simulink model "multi_module_phase_shift_generator_base"  (R2025b)
settings: Solver=FixedStepDiscrete  StartTime=0.0  StopTime=10e3  RelTol=1e-3
settings Model: DataTypeOverride=Off  FPTShortcutValueString='{{},{''BaselineRun_2'',1,1,1,''BaselineRun_2'','''',{},''M'',''F'',''''}}'  Creator=KoayXianCong  LastModifiedBy=KoayXianCong
settings OptimizationCC: BlockReduction=off  ConditionallyExecuteInputs=off  DefaultParameterBehavior=Inlined  InheritOutputTypeSmallerThanSingle=on
settings DebuggingCC: SignalRangeChecking=warning  ArtificialAlgebraicLoopMsg=error  SingleTaskRateTransMsg=error
settings HardwareCC: ProdBitPerPointer=32.0  ProdBitPerSizeT=32.0  ProdBitPerPtrDiffT=32.0  ProdLargestAtomicFloat=None  ProdIntDivRoundTo=Undefined  ProdEndianess=Unspecified  ProdWordSize=32.0  ProdHWDeviceType=ASIC/FPGA->ASIC/FPGA  TargetBitPerPointer=64.0  TargetBitPerSizeT=64.0  TargetBitPerPtrDiffT=64.0  TargetLongLongMode=on  TargetIntDivRoundTo=Zero  TargetEndianess=LittleEndian  TargetWordSize=64.0  TargetHWDeviceType=Custom Processor->MATLAB Host Computer  ProdEqTarget=off

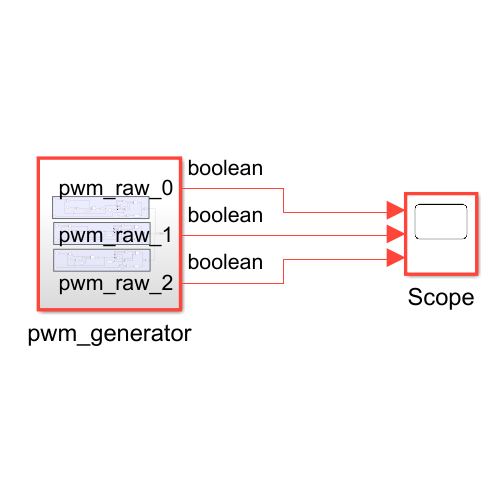
[thumbnail: Simulink's stored preview of the top-level diagram]
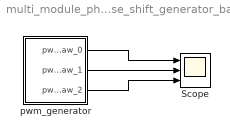
== system multi_module_phase_shift_generator_base ==
  Scope : Scope  NumInputPorts=3
      settings: ActiveDisplayYMinimum=-0.12499999999999997  ActiveDisplayYMaximum=1.125
  pwm_generator : Subsystem
  wires:
  pwm_generator/1(pwm_raw_0) -> Scope/1
  pwm_generator/2(pwm_raw_1) -> Scope/2
  pwm_generator/3(pwm_raw_2) -> Scope/3

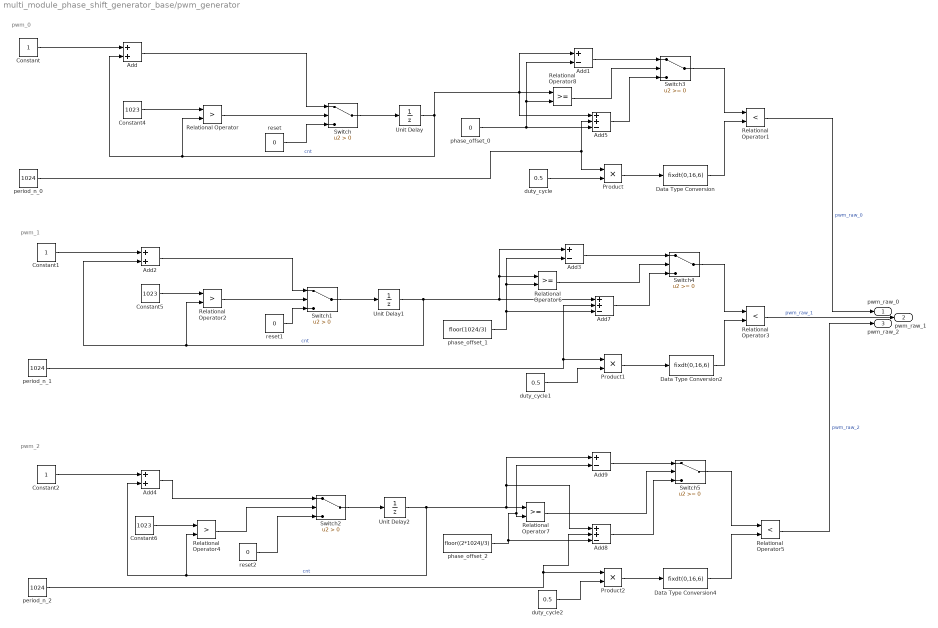
== system multi_module_phase_shift_generator_base/pwm_generator ==
  note: pwm_2
  note: pwm_1
  note: pwm_0
  Add : Sum  OutDataTypeStr=fixdt(0,16,5)
  Add1 : Sum  Inputs=+-
  Add2 : Sum  OutDataTypeStr=fixdt(0,16,5)
  Add3 : Sum  Inputs=+-
  Add4 : Sum  OutDataTypeStr=fixdt(0,16,5)
  Add5 : Sum  Inputs=++-
  Add7 : Sum  Inputs=++-
  Add8 : Sum  Inputs=++-
  Add9 : Sum  Inputs=+-
  Constant : Constant  OutDataTypeStr=fixdt(0,16,15)
  Constant1 : Constant  OutDataTypeStr=fixdt(0,16,15)
  Constant2 : Constant  OutDataTypeStr=fixdt(0,16,15)
  Constant4 : Constant  Value=1023  OutDataTypeStr=uint16  SampleTime=-1
  Constant5 : Constant  Value=1023  OutDataTypeStr=uint16  SampleTime=-1
  Constant6 : Constant  Value=1023  OutDataTypeStr=uint16  SampleTime=-1
  Data Type Conversion : DataTypeConversion  OutDataTypeStr=fixdt(0,16,6)  SaturateOnIntegerOverflow=off  RndMeth=Floor
  Data Type Conversion2 : DataTypeConversion  OutDataTypeStr=fixdt(0,16,6)  SaturateOnIntegerOverflow=off  RndMeth=Floor
  Data Type Conversion4 : DataTypeConversion  OutDataTypeStr=fixdt(0,16,6)  SaturateOnIntegerOverflow=off  RndMeth=Floor
  Product : Product  OutDataTypeStr=fixdt(0,16,6)
  Product1 : Product  OutDataTypeStr=fixdt(0,16,6)
  Product2 : Product  OutDataTypeStr=fixdt(0,16,6)
  Relational Operator : RelationalOperator  Operator=>  OutDataTypeStr=boolean  RndMeth=Simplest  InputSameDT=off
  Relational Operator1 : RelationalOperator  Operator=<  OutDataTypeStr=boolean  RndMeth=Simplest  InputSameDT=off
  Relational Operator2 : RelationalOperator  Operator=>  OutDataTypeStr=boolean  RndMeth=Simplest  InputSameDT=off
  Relational Operator3 : RelationalOperator  Operator=<  OutDataTypeStr=boolean  RndMeth=Simplest  InputSameDT=off
  Relational Operator4 : RelationalOperator  Operator=>  OutDataTypeStr=boolean  RndMeth=Simplest  InputSameDT=off
  Relational Operator5 : RelationalOperator  Operator=<  OutDataTypeStr=boolean  RndMeth=Simplest  InputSameDT=off
  Relational Operator6 : RelationalOperator  OutDataTypeStr=boolean  InputSameDT=off
  Relational Operator7 : RelationalOperator  OutDataTypeStr=boolean  InputSameDT=off
  Relational Operator8 : RelationalOperator  OutDataTypeStr=boolean  InputSameDT=off
  Switch : Switch  Criteria=u2 > Threshold  OutDataTypeStr=fixdt(0,16,5)  SaturateOnIntegerOverflow=off  InputSameDT=off
  Switch1 : Switch  Criteria=u2 > Threshold  OutDataTypeStr=fixdt(0,16,5)  SaturateOnIntegerOverflow=off  InputSameDT=off
  Switch2 : Switch  Criteria=u2 > Threshold  OutDataTypeStr=fixdt(0,16,5)  SaturateOnIntegerOverflow=off  InputSameDT=off
  Switch3 : Switch  SaturateOnIntegerOverflow=off  InputSameDT=off
  Switch4 : Switch  SaturateOnIntegerOverflow=off  InputSameDT=off
  Switch5 : Switch  SaturateOnIntegerOverflow=off  InputSameDT=off
  Unit Delay : UnitDelay  HasFrameUpgradeWarning=on
  Unit Delay1 : UnitDelay  HasFrameUpgradeWarning=on
  Unit Delay2 : UnitDelay  HasFrameUpgradeWarning=on
  duty_cycle : Constant  Value=0.5  OutDataTypeStr=fixdt(0,16,16)
  duty_cycle1 : Constant  Value=0.5  OutDataTypeStr=fixdt(0,16,16)
  duty_cycle2 : Constant  Value=0.5  OutDataTypeStr=fixdt(0,16,16)
  period_n_0 : Constant  Value=1024  OutDataTypeStr=uint16
  period_n_1 : Constant  Value=1024  OutDataTypeStr=uint16
  period_n_2 : Constant  Value=1024  OutDataTypeStr=uint16
  phase_offset_0 : Constant  Value=0  OutDataTypeStr=fixdt(1,16,4)
  phase_offset_1 : Constant  Value=floor(1024/3)  OutDataTypeStr=fixdt(0,16,7)
  phase_offset_2 : Constant  Value=floor((2*1024)/3)  OutDataTypeStr=fixdt(0,16,6)
  reset : Constant  Value=0  OutDataTypeStr=fixdt(1,16,4)
  reset1 : Constant  Value=0  OutDataTypeStr=fixdt(1,16,4)
  reset2 : Constant  Value=0  OutDataTypeStr=fixdt(1,16,4)
  pwm_raw_0 : Outport
  pwm_raw_1 : Outport  Port=2
  pwm_raw_2 : Outport  Port=3
  wires:
  duty_cycle1/1 -> Product1/2
  Switch2/1 -> Unit Delay2/1
  reset2/1 -> Switch2/3
  Relational Operator/1 -> Switch/2
  Product1/1 -> Data Type Conversion2/1
  Data Type Conversion2/1 -> Relational Operator3/2
  reset1/1 -> Switch1/3
  Switch1/1 -> Unit Delay1/1
  Relational Operator4/1 -> Switch2/2
  Unit Delay1/1 -> Relational Operator2/2, Add2/2, Add7/1, Add3/1, Relational Operator6/1  "cnt"
  Add2/1 -> Switch1/1
  Switch5/1 -> Relational Operator5/1
  phase_offset_2/1 -> Add8/3, Add9/2, Relational Operator7/2
  Relational Operator6/1 -> Switch4/2
  Unit Delay/1 -> Add5/1, Add1/1, Relational Operator8/1, Relational Operator/2, Add/2  "cnt"
  Product2/1 -> Data Type Conversion4/1
  phase_offset_1/1 -> Add3/2, Relational Operator6/2, Add7/3
  Data Type Conversion4/1 -> Relational Operator5/2
  period_n_0/1 -> Add5/2, Product/1
  reset/1 -> Switch/3
  Add4/1 -> Switch2/1
  Product/1 -> Data Type Conversion/1
  Unit Delay2/1 -> Add9/1, Add8/1, Relational Operator7/1, Relational Operator4/2, Add4/2  "cnt"
  duty_cycle/1 -> Product/2
  Constant2/1 -> Add4/1
  Relational Operator2/1 -> Switch1/2
  duty_cycle2/1 -> Product2/2
  Constant1/1 -> Add2/1
  period_n_2/1 -> Add8/2, Product2/1
  Switch4/1 -> Relational Operator3/1
  Relational Operator5/1 -> pwm_raw_2/1  "pwm_raw_2"
  Switch/1 -> Unit Delay/1
  Add/1 -> Switch/1
  Constant/1 -> Add/1
  Switch3/1 -> Relational Operator1/1
  Relational Operator3/1 -> pwm_raw_1/1  "pwm_raw_1"
  Data Type Conversion/1 -> Relational Operator1/2
  phase_offset_0/1 -> Add1/2, Relational Operator8/2, Add5/3
  Constant4/1 -> Relational Operator/1
  Constant5/1 -> Relational Operator2/1
  Constant6/1 -> Relational Operator4/1
  Relational Operator1/1 -> pwm_raw_0/1  "pwm_raw_0"
  period_n_1/1 -> Add7/2, Product1/1
  Add3/1 -> Switch4/1
  Add7/1 -> Switch4/3
  Add9/1 -> Switch5/1
  Relational Operator7/1 -> Switch5/2
  Add8/1 -> Switch5/3
  Add5/1 -> Switch3/3
  Add1/1 -> Switch3/1
  Relational Operator8/1 -> Switch3/2
